simulink model "s1019a"  (Simulink 6.0)
settings: Solver=ode3  SolverMode=SingleTasking  StartTime=0.0  StopTime=900  FixedStep=1  MaxStep=1  RelTol=1e-3  AbsTol=1e-3
values from neighbouring files (symbols this model uses):
  wdach = 0    [m0109b.m]    (also in m0404Bsp.m = 1)
  zdach = -.3    (= -0.3)    [m0109b.m]    (also in m0404Bsp.m = 1)
undefined symbols (not defined in the file or in its folder): steptime
settings Model: LastModifiedBy=Froriep
settings DataIOCC: LimitDataPoints=off  SaveOutput=off  TimeSaveName=t
settings OptimizationCC: BooleanDataType=off
settings DebuggingCC: SolverPrmCheckMsg=none
settings HardwareCC: TargetUnknown=on
settings STFCustomTargetCC: TargetFcnLib=ansi_tfl_tmw.mat  GenFloatMathFcnCalls=ANSI_C  ModelReferenceCompliant=off  SystemTargetFile=grt.tlc

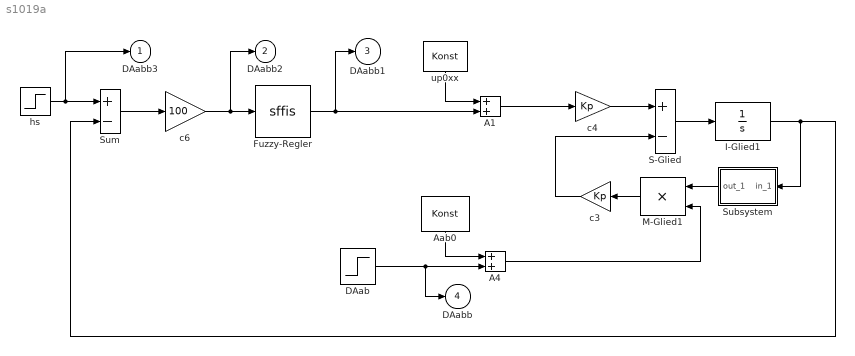
== system s1019a ==
  A1 : Sum  SaturateOnIntegerOverflow=on  InputSameDT=on
  A4 : Sum  SaturateOnIntegerOverflow=on  InputSameDT=on
  Aab0 : Constant  Orientation=down  Value=Konst  mask(Konstante){@1=Aab0}
      mask prompts: @1 "Wert"
      mask help: Konstante
      mask init:
      | Konst=@1;
      mask Display: disp('Aab0')
  DAab : Step  Time=steptime  After=zdach  SampleTime=0
  Fuzzy-Regler : S-Function  FunctionName=sffis  Parameters=fismatrix  mask(FIS){@1=fuell}
      mask prompts: @1 "FIS Matrix:"
      mask help: FIS
      mask init:
      | fismatrix = @1;
      mask Help: Fuzzy Inference System
      mask Display: plot(0, -0.3, 6, -0.3, 0, 1.2, 6, 1.2, [0 6], [0 0], [1 2 3],[0 1 0],[2 3 4],[0 1 0],[3 4 5],[0 1 0])
  I-Glied1 : Integrator  InitialCondition=x0  mask(I-Glied){@1=hs}
      mask prompts: @1 "Anfangswert"
      mask help: I-Glied
      mask init:
      | x0=@1;
      mask Display: disp('I-Glied')
  M-Glied1 : Product  Orientation=left  SaturateOnIntegerOverflow=on  RndMeth=Zero  InputSameDT=on
  S-Glied : Sum  Inputs=+-  SaturateOnIntegerOverflow=on  InputSameDT=on
  Subsystem : Subsystem  Orientation=left
      mask Display: disp('Wurzel')
  Sum : Sum  Inputs=+-  SaturateOnIntegerOverflow=on  InputSameDT=on
  c3 : Gain  Orientation=left  Gain=Kp  SaturateOnIntegerOverflow=on  mask(P-Glied){@1=c1}
      mask prompts: @1 "Beiwert"
      mask help: P-Glied
      mask init:
      | Kp=@1;
      mask Display: disp('c1')
  c4 : Gain  Gain=Kp  SaturateOnIntegerOverflow=on  mask(P-Glied){@1=c2}
      mask prompts: @1 "Beiwert"
      mask help: P-Glied
      mask init:
      | Kp=@1;
      mask Display: disp('c2')
  c6 : Gain  Gain=100  SaturateOnIntegerOverflow=on
      mask Display: disp('K')
  hs : Step  Time=0  After=wdach  SampleTime=0
  up0xx : Constant  Orientation=down  Value=Konst  mask(Konstante){@1=up0}
      mask prompts: @1 "Wert"
      mask help: Konstante
      mask init:
      | Konst=@1;
      mask Display: disp('up0')
  DAabb3 : Outport  InitialOutput=0
  DAabb2 : Outport  Port=2  InitialOutput=0
  DAabb1 : Outport  Port=3  InitialOutput=0
  DAabb : Outport  Port=4  InitialOutput=0
  wires:
  DAab/1 -> A4/2, DAabb/1
  c4/1 -> S-Glied/1
  S-Glied/1 -> I-Glied1/1
  M-Glied1/1 -> c3/1
  Subsystem/1(out_1) -> M-Glied1/1
  c3/1 -> S-Glied/2
  A4/1 -> M-Glied1/2
  A1/1 -> c4/1
  Aab0/1 -> A4/1
  Fuzzy-Regler/1 -> A1/2, DAabb1/1
  Sum/1 -> c6/1
  c6/1 -> Fuzzy-Regler/1, DAabb2/1
  up0xx/1 -> A1/1
  I-Glied1/1 -> Subsystem/1(in_1), Sum/2
  hs/1 -> Sum/1, DAabb3/1

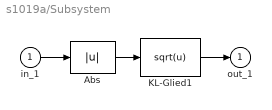
== system s1019a/Subsystem ==
  in_1 : Inport  Port=1  LatchInput=off
  Abs : Abs  SaturateOnIntegerOverflow=on
  KL-Glied1 : Fcn  Expr=sqrt(u)
  out_1 : Outport  InitialOutput=0
  wires:
  Abs/1 -> KL-Glied1/1
  in_1/1 -> Abs/1
  KL-Glied1/1 -> out_1/1
